simulink model "Rotary_Encoder"  (R2019a)
settings: Solver=VariableStepAuto  StartTime=0.0  StopTime=10.0  RelTol=1e-3
model workspace (MAT data in the model file):
  L = 180
settings Model: Creator=Saif Qadeer  LastModifiedBy=Saif Qadeer

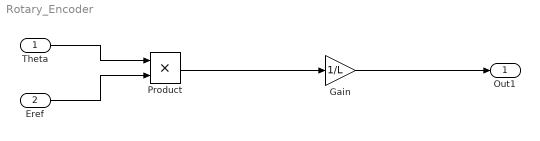
== system Rotary_Encoder ==
  Theta : Inport
  Eref : Inport  Port=2
  Gain : Gain  Gain=1/L
  Product : Product
  Out1 : Outport
  wires:
  Gain/1 -> Out1/1
  Theta/1 -> Product/1
  Eref/1 -> Product/2
  Product/1 -> Gain/1
